simulink model "PTTransmCU"  (Simulink 7.7)
settings: Solver=ode45  StartTime=0.0  StopTime=inf  RelTol=1e-3
libraries: simulink x3, CarMaker4SL x2
(part 2 of 2)

== system PTTransmCU/CarMaker/IPG Vehicle/CarAndTrailer/Trailer/CreateBus Vhcl.Wheel.FR ==
  In1 : Inport
  Bus Creator3 : BusCreator  Inputs=14
  Demux3 : Demux  Outputs=14
  Out1 : Outport
  wires:
  Demux3/1 -> Bus Creator3/1  "Vhcl Wheel FR t x"
  Bus Creator3/1 -> Out1/1
  In1/1 -> Demux3/1
  Demux3/2 -> Bus Creator3/2  "Vhcl Wheel FR t y"
  Demux3/3 -> Bus Creator3/3  "Vhcl Wheel FR t z"
  Demux3/4 -> Bus Creator3/4  "Vhcl Wheel FR r_zxy x"
  Demux3/5 -> Bus Creator3/5  "Vhcl Wheel FR r_zxy y"
  Demux3/6 -> Bus Creator3/6  "Vhcl Wheel FR r_zxy z"
  Demux3/7 -> Bus Creator3/7  "Vhcl Wheel FR Fx"
  Demux3/8 -> Bus Creator3/8  "Vhcl Wheel FR Fy"
  Demux3/9 -> Bus Creator3/9  "Vhcl Wheel FR Fz"
  Demux3/10 -> Bus Creator3/10  "Vhcl Wheel FR vBelt"
  Demux3/11 -> Bus Creator3/11  "Vhcl Wheel FR LongSlip"
  Demux3/12 -> Bus Creator3/12  "Vhcl Wheel FR SideSlip"
  Demux3/13 -> Bus Creator3/13  "Vhcl Wheel FR Trq_T2W"
  Demux3/14 -> Bus Creator3/14  "Vhcl Wheel FR Trq_WhlBearing"

== system PTTransmCU/CarMaker/IPG Vehicle/CarAndTrailer/Trailer/CreateBus Vhcl.Wheel.RL ==
  In1 : Inport
  Bus Creator3 : BusCreator  Inputs=14
  Demux3 : Demux  Outputs=14
  Out1 : Outport
  wires:
  Demux3/1 -> Bus Creator3/1  "Vhcl Wheel RL t x"
  Bus Creator3/1 -> Out1/1
  In1/1 -> Demux3/1
  Demux3/2 -> Bus Creator3/2  "Vhcl Wheel RL t y"
  Demux3/3 -> Bus Creator3/3  "Vhcl Wheel RL t z"
  Demux3/4 -> Bus Creator3/4  "Vhcl Wheel RL r_zxy x"
  Demux3/5 -> Bus Creator3/5  "Vhcl Wheel RL r_zxy y"
  Demux3/6 -> Bus Creator3/6  "Vhcl Wheel RL r_zxy z"
  Demux3/7 -> Bus Creator3/7  "Vhcl Wheel RL Fx"
  Demux3/8 -> Bus Creator3/8  "Vhcl Wheel RL Fy"
  Demux3/9 -> Bus Creator3/9  "Vhcl Wheel RL Fz"
  Demux3/10 -> Bus Creator3/10  "Vhcl Wheel RL vBelt"
  Demux3/11 -> Bus Creator3/11  "Vhcl Wheel RL LongSlip"
  Demux3/12 -> Bus Creator3/12  "Vhcl Wheel RL SideSlip"
  Demux3/13 -> Bus Creator3/13  "Vhcl Wheel RL Trq_T2W"
  Demux3/14 -> Bus Creator3/14  "Vhcl Wheel RL Trq_WhlBearing"

== system PTTransmCU/CarMaker/IPG Vehicle/CarAndTrailer/Trailer/CreateBus Vhcl.Wheel.RR ==
  In1 : Inport
  Bus Creator3 : BusCreator  Inputs=14
  Demux3 : Demux  Outputs=14
  Out1 : Outport
  wires:
  Demux3/1 -> Bus Creator3/1  "Vhcl Wheel RR t x"
  Bus Creator3/1 -> Out1/1
  In1/1 -> Demux3/1
  Demux3/2 -> Bus Creator3/2  "Vhcl Wheel RR t y"
  Demux3/3 -> Bus Creator3/3  "Vhcl Wheel RR t z"
  Demux3/4 -> Bus Creator3/4  "Vhcl Wheel RR r_zxy x"
  Demux3/5 -> Bus Creator3/5  "Vhcl Wheel RR r_zxy y"
  Demux3/6 -> Bus Creator3/6  "Vhcl Wheel RR r_zxy z"
  Demux3/7 -> Bus Creator3/7  "Vhcl Wheel RR Fx"
  Demux3/8 -> Bus Creator3/8  "Vhcl Wheel RR Fy"
  Demux3/9 -> Bus Creator3/9  "Vhcl Wheel RR Fz"
  Demux3/10 -> Bus Creator3/10  "Vhcl Wheel RR vBelt"
  Demux3/11 -> Bus Creator3/11  "Vhcl Wheel RR LongSlip"
  Demux3/12 -> Bus Creator3/12  "Vhcl Wheel RR SideSlip"
  Demux3/13 -> Bus Creator3/13  "Vhcl Wheel RR Trq_T2W"
  Demux3/14 -> Bus Creator3/14  "Vhcl Wheel RR Trq_WhlBearing"

== system PTTransmCU/CarMaker/IPG Vehicle/PowerTrain/TCU Example/CreateBus TCU ClutchOut ==
  In : Inport
  BusCreator : BusCreator  Inputs=1
  Demux : Demux  Outputs=1
  Out : Outport
  wires:
  In/1 -> Demux/1
  BusCreator/1 -> Out/1
  Demux/1 -> BusCreator/1  "TCU ClutchOut Pos"

== system PTTransmCU/CarMaker/IPG Vehicle/PowerTrain/TCU Example/CreateBus TCU GearBoxM_Out0 ==
  In : Inport
  BusCreator : BusCreator
  Demux : Demux
  Out : Outport
  wires:
  In/1 -> Demux/1
  BusCreator/1 -> Out/1
  Demux/1 -> BusCreator/1  "TCU GearBoxM_Out0 GearNoTrg"
  Demux/2 -> BusCreator/2  "TCU GearBoxM_Out0 set_ParkBrake"
  Demux/3 -> BusCreator/3  "TCU GearBoxM_Out0 Trq_in_off"
  Demux/4 -> BusCreator/4  "TCU GearBoxM_Out0 Clutch Pos"

== system PTTransmCU/CarMaker/IPG Vehicle/PowerTrain/TCU Example/CreateBus TCU GearBoxM_Out1 ==
  In : Inport
  BusCreator : BusCreator
  Demux : Demux
  Out : Outport
  wires:
  In/1 -> Demux/1
  BusCreator/1 -> Out/1
  Demux/1 -> BusCreator/1  "TCU GearBoxM_Out1 GearNoTrg"
  Demux/2 -> BusCreator/2  "TCU GearBoxM_Out1 set_ParkBrake"
  Demux/3 -> BusCreator/3  "TCU GearBoxM_Out1 Trq_in_off"
  Demux/4 -> BusCreator/4  "TCU GearBoxM_Out1 Clutch Pos"

== system PTTransmCU/CarMaker/IPG Vehicle/PowerTrain/TCU Example/CreateBus TCU GearBoxM_Out2 ==
  In : Inport
  BusCreator : BusCreator
  Demux : Demux
  Out : Outport
  wires:
  In/1 -> Demux/1
  BusCreator/1 -> Out/1
  Demux/1 -> BusCreator/1  "TCU GearBoxM_Out2 GearNoTrg"
  Demux/2 -> BusCreator/2  "TCU GearBoxM_Out2 set_ParkBrake"
  Demux/3 -> BusCreator/3  "TCU GearBoxM_Out2 Trq_in_off"
  Demux/4 -> BusCreator/4  "TCU GearBoxM_Out2 Clutch Pos"

== system PTTransmCU/CarMaker/IPG Vehicle/PowerTrain/TCU Example/CreateBus TCU GearBoxM_Out3 ==
  In : Inport
  BusCreator : BusCreator
  Demux : Demux
  Out : Outport
  wires:
  In/1 -> Demux/1
  BusCreator/1 -> Out/1
  Demux/1 -> BusCreator/1  "TCU GearBoxM_Out3 GearNoTrg"
  Demux/2 -> BusCreator/2  "TCU GearBoxM_Out3 set_ParkBrake"
  Demux/3 -> BusCreator/3  "TCU GearBoxM_Out3 Trq_in_off"
  Demux/4 -> BusCreator/4  "TCU GearBoxM_Out3 Clutch Pos"

== system PTTransmCU/CarMaker/IPG Vehicle/PowerTrain/TCU Example/CreateBus TCU GearBoxOut ==
  In : Inport
  BusCreator : BusCreator
  Demux : Demux
  Out : Outport
  wires:
  In/1 -> Demux/1
  BusCreator/1 -> Out/1
  Demux/1 -> BusCreator/1  "TCU GearBoxOut GearNoTrg"
  Demux/2 -> BusCreator/2  "TCU GearBoxOut set_ParkBrake"
  Demux/3 -> BusCreator/3  "TCU GearBoxOut Trq_in_off"
  Demux/4 -> BusCreator/4  "TCU GearBoxOut Clutch Pos"

== system PTTransmCU/CarMaker/IPG Vehicle/PowerTrain/TCU Example/CreateBus TCU Status ==
  In : Inport
  BusCreator : BusCreator  Inputs=1
  Demux : Demux  Outputs=1
  Out : Outport
  wires:
  In/1 -> Demux/1
  BusCreator/1 -> Out/1
  Demux/1 -> BusCreator/1  "TCU_Out Status"

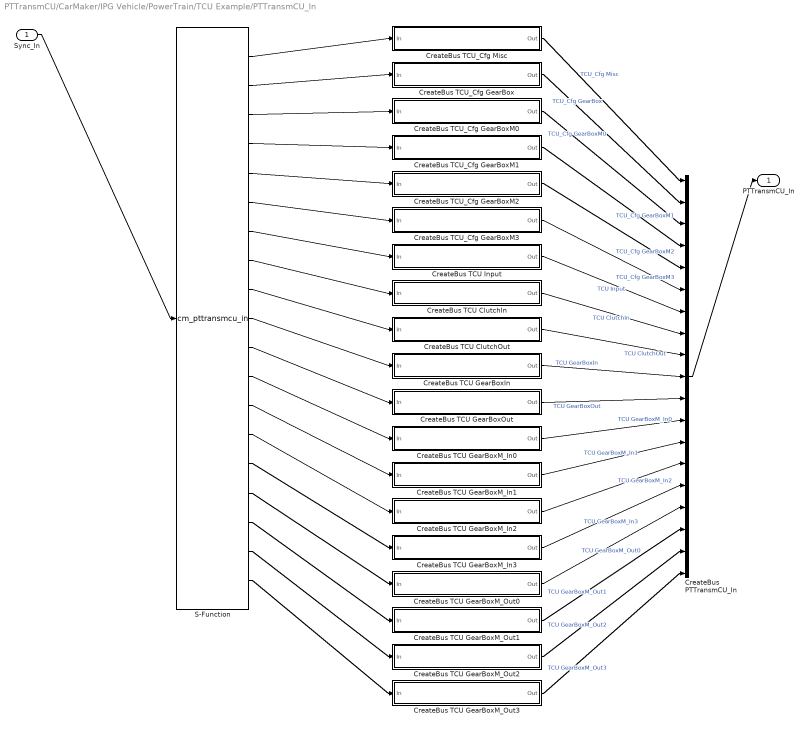
== system PTTransmCU/CarMaker/IPG Vehicle/PowerTrain/TCU Example/PTTransmCU_In ==
  Sync_In : Inport
  CreateBus PTTransmCU_In : BusCreator  Inputs=19
  CreateBus TCU ClutchIn : Subsystem
  CreateBus TCU ClutchOut : Subsystem
  CreateBus TCU GearBoxIn : Subsystem
  CreateBus TCU GearBoxM_In0 : Subsystem
  CreateBus TCU GearBoxM_In1 : Subsystem
  CreateBus TCU GearBoxM_In2 : Subsystem
  CreateBus TCU GearBoxM_In3 : Subsystem
  CreateBus TCU GearBoxM_Out0 : Subsystem
  CreateBus TCU GearBoxM_Out1 : Subsystem
  CreateBus TCU GearBoxM_Out2 : Subsystem
  CreateBus TCU GearBoxM_Out3 : Subsystem
  CreateBus TCU GearBoxOut : Subsystem
  CreateBus TCU Input : Subsystem
  CreateBus TCU_Cfg GearBox : Subsystem
  CreateBus TCU_Cfg GearBoxM0 : Subsystem
  CreateBus TCU_Cfg GearBoxM1 : Subsystem
  CreateBus TCU_Cfg GearBoxM2 : Subsystem
  CreateBus TCU_Cfg GearBoxM3 : Subsystem
  CreateBus TCU_Cfg Misc : Subsystem
  S-Function : S-Function  FunctionName=cm_pttransmcu_in  EnableBusSupport=off
  PTTransmCU_In : Outport
  wires:
  Sync_In/1 -> S-Function/1
  CreateBus PTTransmCU_In/1 -> PTTransmCU_In/1
  S-Function/1 -> CreateBus TCU_Cfg Misc/1(In)
  CreateBus TCU_Cfg Misc/1(Out) -> CreateBus PTTransmCU_In/1  "TCU_Cfg Misc"
  S-Function/2 -> CreateBus TCU_Cfg GearBox/1(In)
  CreateBus TCU_Cfg GearBox/1(Out) -> CreateBus PTTransmCU_In/2  "TCU_Cfg GearBox"
  S-Function/3 -> CreateBus TCU_Cfg GearBoxM0/1(In)
  CreateBus TCU_Cfg GearBoxM0/1(Out) -> CreateBus PTTransmCU_In/3  "TCU_Cfg GearBoxM0"
  S-Function/4 -> CreateBus TCU_Cfg GearBoxM1/1(In)
  CreateBus TCU_Cfg GearBoxM1/1(Out) -> CreateBus PTTransmCU_In/4  "TCU_Cfg GearBoxM1"
  S-Function/5 -> CreateBus TCU_Cfg GearBoxM2/1(In)
  CreateBus TCU_Cfg GearBoxM2/1(Out) -> CreateBus PTTransmCU_In/5  "TCU_Cfg GearBoxM2"
  S-Function/6 -> CreateBus TCU_Cfg GearBoxM3/1(In)
  CreateBus TCU_Cfg GearBoxM3/1(Out) -> CreateBus PTTransmCU_In/6  "TCU_Cfg GearBoxM3"
  S-Function/7 -> CreateBus TCU Input/1(In)
  CreateBus TCU Input/1(Out) -> CreateBus PTTransmCU_In/7  "TCU Input"
  S-Function/8 -> CreateBus TCU ClutchIn/1(In)
  CreateBus TCU ClutchIn/1(Out) -> CreateBus PTTransmCU_In/8  "TCU ClutchIn"
  S-Function/9 -> CreateBus TCU ClutchOut/1(In)
  CreateBus TCU ClutchOut/1(Out) -> CreateBus PTTransmCU_In/9  "TCU ClutchOut"
  S-Function/10 -> CreateBus TCU GearBoxIn/1(In)
  CreateBus TCU GearBoxIn/1(Out) -> CreateBus PTTransmCU_In/10  "TCU GearBoxIn"
  S-Function/11 -> CreateBus TCU GearBoxOut/1(In)
  CreateBus TCU GearBoxOut/1(Out) -> CreateBus PTTransmCU_In/11  "TCU GearBoxOut"
  S-Function/12 -> CreateBus TCU GearBoxM_In0/1(In)
  CreateBus TCU GearBoxM_In0/1(Out) -> CreateBus PTTransmCU_In/12  "TCU GearBoxM_In0"
  S-Function/13 -> CreateBus TCU GearBoxM_In1/1(In)
  CreateBus TCU GearBoxM_In1/1(Out) -> CreateBus PTTransmCU_In/13  "TCU GearBoxM_In1"
  S-Function/14 -> CreateBus TCU GearBoxM_In2/1(In)
  CreateBus TCU GearBoxM_In2/1(Out) -> CreateBus PTTransmCU_In/14  "TCU GearBoxM_In2"
  S-Function/15 -> CreateBus TCU GearBoxM_In3/1(In)
  CreateBus TCU GearBoxM_In3/1(Out) -> CreateBus PTTransmCU_In/15  "TCU GearBoxM_In3"
  S-Function/16 -> CreateBus TCU GearBoxM_Out0/1(In)
  CreateBus TCU GearBoxM_Out0/1(Out) -> CreateBus PTTransmCU_In/16  "TCU GearBoxM_Out0"
  S-Function/17 -> CreateBus TCU GearBoxM_Out1/1(In)
  CreateBus TCU GearBoxM_Out1/1(Out) -> CreateBus PTTransmCU_In/17  "TCU GearBoxM_Out1"
  S-Function/18 -> CreateBus TCU GearBoxM_Out2/1(In)
  CreateBus TCU GearBoxM_Out2/1(Out) -> CreateBus PTTransmCU_In/18  "TCU GearBoxM_Out2"
  S-Function/19 -> CreateBus TCU GearBoxM_Out3/1(In)
  CreateBus TCU GearBoxM_Out3/1(Out) -> CreateBus PTTransmCU_In/19  "TCU GearBoxM_Out3"

== system PTTransmCU/CarMaker/IPG Vehicle/PowerTrain/TCU Example/PTTransmCU_Out ==
  TCU Status : Inport
  TCU ClutchOut : Inport  Port=2
  TCU GearBoxOut : Inport  Port=3
  TCU GearBoxM_Out0 : Inport  Port=4
  TCU GearBoxM_Out1 : Inport  Port=5
  TCU GearBoxM_Out2 : Inport  Port=6
  TCU GearBoxM_Out3 : Inport  Port=7
  S-Function : S-Function  FunctionName=cm_pttransmcu_out  EnableBusSupport=off
  wires:
  TCU Status/1 -> S-Function/1
  TCU ClutchOut/1 -> S-Function/2
  TCU GearBoxOut/1 -> S-Function/3
  TCU GearBoxM_Out0/1 -> S-Function/4
  TCU GearBoxM_Out1/1 -> S-Function/5
  TCU GearBoxM_Out2/1 -> S-Function/6
  TCU GearBoxM_Out3/1 -> S-Function/7

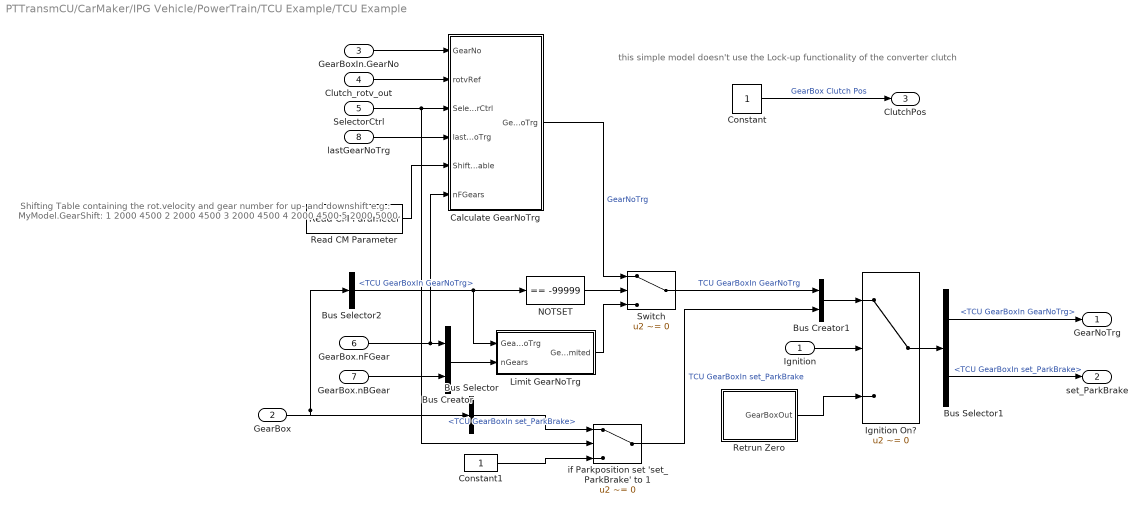
== system PTTransmCU/CarMaker/IPG Vehicle/PowerTrain/TCU Example/TCU Example ==
  note: this simple model doesn't use the
      | Lock-up functionality of the converter clutch
  note: Shifting Table containing the rot.velocity
      | and gear number for up- and downshift
      | e.g.:
      | MyModel.GearShift:
      |     1    2000    4500
      |     2    2000    4500
      |     3    2000    4500
      |     4    2000    4500
      |     5    2000    5000
  Ignition : Inport
  GearBox : Inport  Port=2
  GearBoxIn.GearNo : Inport  Port=3
  Clutch_rotv_out : Inport  Port=4
  SelectorCtrl : Inport  Port=5
  GearBox.nFGear : Inport  Port=6
  GearBox.nBGear : Inport  Port=7
  lastGearNoTrg : Inport  Port=8
  Bus Creator : BusCreator  Inputs=2
  Bus Creator1 : BusCreator  Inputs=2
  Bus Selector : BusSelector  OutputSignals=TCU GearBoxIn set_ParkBrake
  Bus Selector1 : BusSelector  OutputSignals=TCU GearBoxIn GearNoTrg,TCU GearBoxIn set_ParkBrake
  Bus Selector2 : BusSelector  OutputSignals=TCU GearBoxIn GearNoTrg
  Calculate GearNoTrg : Subsystem  TreatAsAtomicUnit=on
  Constant : Constant
  Constant1 : Constant
  Ignition On? : Switch  Criteria=u2 ~= 0
  Limit GearNoTrg : Subsystem
  NOTSET : simulink/Logic and Bit Operations/Compare To Constant  SystemSampleTime=-1  relop===  const=-99999  LogicOutDataTypeMode=uint8
  Read CM Parameter : CarMaker4SL/Read CM Parameter  xfile=Vehicle  xkey=MyModel.GearShift  xnout=80  xdefaults=0  xmuxed=on
  Retrun Zero : Subsystem  TreatAsAtomicUnit=on
  Switch : Switch  Criteria=u2 ~= 0
  if Parkposition set 'set_ParkBrake' to 1 : Switch  Criteria=u2 ~= 0
  GearNoTrg : Outport
  set_ParkBrake : Outport  Port=2
  ClutchPos : Outport  Port=3
  wires:
  GearBox/1 -> Bus Selector2/1, Bus Selector/1
  GearBox.nFGear/1 -> Bus Creator/1, Calculate GearNoTrg/6(nFGears)
  GearBoxIn.GearNo/1 -> Calculate GearNoTrg/1(GearNo)
  Constant/1 -> ClutchPos/1  "GearBox Clutch Pos"
  NOTSET/1 -> Switch/2
  Bus Selector2/1 -> Limit GearNoTrg/1(GearNoTrg), NOTSET/1  "<TCU GearBoxIn GearNoTrg>"
  Bus Creator/1 -> Limit GearNoTrg/2(nGears)
  Ignition/1 -> Ignition On?/2
  Clutch_rotv_out/1 -> Calculate GearNoTrg/2(rotvRef)
  SelectorCtrl/1 -> Calculate GearNoTrg/3(SelectorCtrl), if Parkposition set 'set_ParkBrake' to 1/2
  Read CM Parameter/1 -> Calculate GearNoTrg/5(ShiftingTable)
  Bus Creator1/1 -> Ignition On?/1
  Switch/1 -> Bus Creator1/1  "TCU GearBoxIn GearNoTrg"
  Calculate GearNoTrg/1(GearNoTrg) -> Switch/1  "GearNoTrg"
  Limit GearNoTrg/1(GearNoTrg_limited) -> Switch/3
  lastGearNoTrg/1 -> Calculate GearNoTrg/4(lastGearNoTrg)
  GearBox.nBGear/1 -> Bus Creator/2
  Bus Selector1/1 -> GearNoTrg/1  "<TCU GearBoxIn GearNoTrg>"
  Bus Selector1/2 -> set_ParkBrake/1  "<TCU GearBoxIn set_ParkBrake>"
  Retrun Zero/1(GearBoxOut) -> Ignition On?/3
  Ignition On?/1 -> Bus Selector1/1
  if Parkposition set 'set_ParkBrake' to 1/1 -> Bus Creator1/2  "TCU GearBoxIn set_ParkBrake"
  Bus Selector/1 -> if Parkposition set 'set_ParkBrake' to 1/1  "<TCU GearBoxIn set_ParkBrake>"
  Constant1/1 -> if Parkposition set 'set_ParkBrake' to 1/3

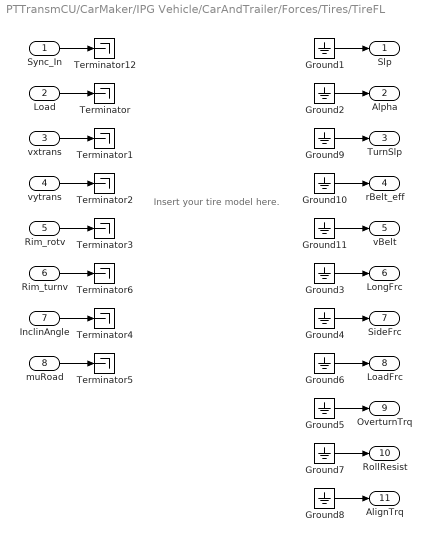
== system PTTransmCU/CarMaker/IPG Vehicle/CarAndTrailer/Forces/Tires/TireFL ==
  note: Insert your tire model here.
  Sync_In : Inport
  Load : Inport  Port=2
  vxtrans : Inport  Port=3
  vytrans : Inport  Port=4
  Rim_rotv : Inport  Port=5
  Rim_turnv : Inport  Port=6
  InclinAngle : Inport  Port=7
  muRoad : Inport  Port=8
  Ground{1..11} (11 alike) : Ground
  Terminator{,1..6,12} (8 alike) : Terminator
  Slp : Outport
  Alpha : Outport  Port=2
  TurnSlp : Outport  Port=3
  rBelt_eff : Outport  Port=4
  vBelt : Outport  Port=5
  LongFrc : Outport  Port=6
  SideFrc : Outport  Port=7
  LoadFrc : Outport  Port=8
  OverturnTrq : Outport  Port=9
  RollResist : Outport  Port=10
  AlignTrq : Outport  Port=11
  wires:
  Ground11/1 -> vBelt/1
  Ground10/1 -> rBelt_eff/1
  Ground9/1 -> TurnSlp/1
  Rim_turnv/1 -> Terminator6/1
  Sync_In/1 -> Terminator12/1
  Ground2/1 -> Alpha/1
  Ground3/1 -> LongFrc/1
  Ground4/1 -> SideFrc/1
  Ground5/1 -> OverturnTrq/1
  vxtrans/1 -> Terminator1/1
  vytrans/1 -> Terminator2/1
  Rim_rotv/1 -> Terminator3/1
  InclinAngle/1 -> Terminator4/1
  muRoad/1 -> Terminator5/1
  Load/1 -> Terminator/1
  Ground1/1 -> Slp/1
  Ground6/1 -> LoadFrc/1
  Ground7/1 -> RollResist/1
  Ground8/1 -> AlignTrq/1

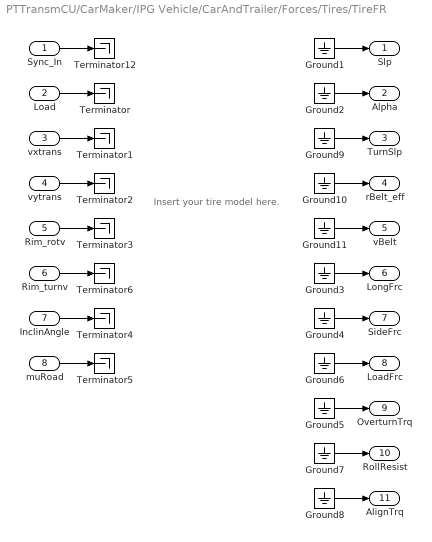
== system PTTransmCU/CarMaker/IPG Vehicle/CarAndTrailer/Forces/Tires/TireFR ==
  note: Insert your tire model here.
  Sync_In : Inport
  Load : Inport  Port=2
  vxtrans : Inport  Port=3
  vytrans : Inport  Port=4
  Rim_rotv : Inport  Port=5
  Rim_turnv : Inport  Port=6
  InclinAngle : Inport  Port=7
  muRoad : Inport  Port=8
  Ground{1..11} (11 alike) : Ground
  Terminator{,1..6,12} (8 alike) : Terminator
  Slp : Outport
  Alpha : Outport  Port=2
  TurnSlp : Outport  Port=3
  rBelt_eff : Outport  Port=4
  vBelt : Outport  Port=5
  LongFrc : Outport  Port=6
  SideFrc : Outport  Port=7
  LoadFrc : Outport  Port=8
  OverturnTrq : Outport  Port=9
  RollResist : Outport  Port=10
  AlignTrq : Outport  Port=11
  wires:
  Ground11/1 -> vBelt/1
  Ground10/1 -> rBelt_eff/1
  Ground9/1 -> TurnSlp/1
  Rim_turnv/1 -> Terminator6/1
  Sync_In/1 -> Terminator12/1
  Ground2/1 -> Alpha/1
  Ground3/1 -> LongFrc/1
  Ground4/1 -> SideFrc/1
  Ground5/1 -> OverturnTrq/1
  vxtrans/1 -> Terminator1/1
  vytrans/1 -> Terminator2/1
  Rim_rotv/1 -> Terminator3/1
  InclinAngle/1 -> Terminator4/1
  muRoad/1 -> Terminator5/1
  Load/1 -> Terminator/1
  Ground1/1 -> Slp/1
  Ground6/1 -> LoadFrc/1
  Ground7/1 -> RollResist/1
  Ground8/1 -> AlignTrq/1

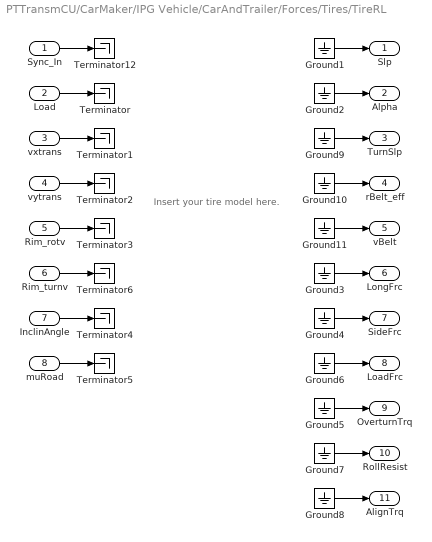
== system PTTransmCU/CarMaker/IPG Vehicle/CarAndTrailer/Forces/Tires/TireRL ==
  note: Insert your tire model here.
  Sync_In : Inport
  Load : Inport  Port=2
  vxtrans : Inport  Port=3
  vytrans : Inport  Port=4
  Rim_rotv : Inport  Port=5
  Rim_turnv : Inport  Port=6
  InclinAngle : Inport  Port=7
  muRoad : Inport  Port=8
  Ground{1..11} (11 alike) : Ground
  Terminator{,1..6,12} (8 alike) : Terminator
  Slp : Outport
  Alpha : Outport  Port=2
  TurnSlp : Outport  Port=3
  rBelt_eff : Outport  Port=4
  vBelt : Outport  Port=5
  LongFrc : Outport  Port=6
  SideFrc : Outport  Port=7
  LoadFrc : Outport  Port=8
  OverturnTrq : Outport  Port=9
  RollResist : Outport  Port=10
  AlignTrq : Outport  Port=11
  wires:
  Ground11/1 -> vBelt/1
  Ground10/1 -> rBelt_eff/1
  Ground9/1 -> TurnSlp/1
  Rim_turnv/1 -> Terminator6/1
  Sync_In/1 -> Terminator12/1
  Ground2/1 -> Alpha/1
  Ground3/1 -> LongFrc/1
  Ground4/1 -> SideFrc/1
  Ground5/1 -> OverturnTrq/1
  vxtrans/1 -> Terminator1/1
  vytrans/1 -> Terminator2/1
  Rim_rotv/1 -> Terminator3/1
  InclinAngle/1 -> Terminator4/1
  muRoad/1 -> Terminator5/1
  Load/1 -> Terminator/1
  Ground1/1 -> Slp/1
  Ground6/1 -> LoadFrc/1
  Ground7/1 -> RollResist/1
  Ground8/1 -> AlignTrq/1

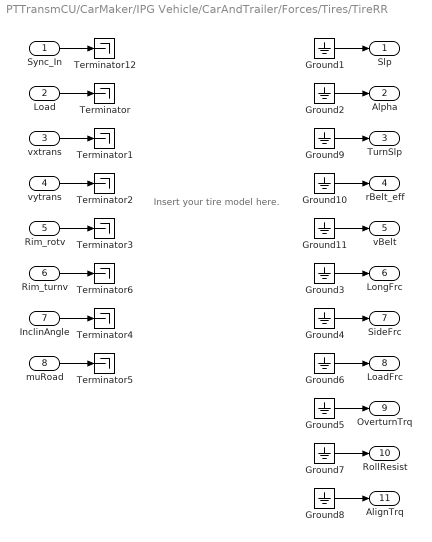
== system PTTransmCU/CarMaker/IPG Vehicle/CarAndTrailer/Forces/Tires/TireRR ==
  note: Insert your tire model here.
  Sync_In : Inport
  Load : Inport  Port=2
  vxtrans : Inport  Port=3
  vytrans : Inport  Port=4
  Rim_rotv : Inport  Port=5
  Rim_turnv : Inport  Port=6
  InclinAngle : Inport  Port=7
  muRoad : Inport  Port=8
  Ground{1..11} (11 alike) : Ground
  Terminator{,1..6,12} (8 alike) : Terminator
  Slp : Outport
  Alpha : Outport  Port=2
  TurnSlp : Outport  Port=3
  rBelt_eff : Outport  Port=4
  vBelt : Outport  Port=5
  LongFrc : Outport  Port=6
  SideFrc : Outport  Port=7
  LoadFrc : Outport  Port=8
  OverturnTrq : Outport  Port=9
  RollResist : Outport  Port=10
  AlignTrq : Outport  Port=11
  wires:
  Ground11/1 -> vBelt/1
  Ground10/1 -> rBelt_eff/1
  Ground9/1 -> TurnSlp/1
  Rim_turnv/1 -> Terminator6/1
  Sync_In/1 -> Terminator12/1
  Ground2/1 -> Alpha/1
  Ground3/1 -> LongFrc/1
  Ground4/1 -> SideFrc/1
  Ground5/1 -> OverturnTrq/1
  vxtrans/1 -> Terminator1/1
  vytrans/1 -> Terminator2/1
  Rim_rotv/1 -> Terminator3/1
  InclinAngle/1 -> Terminator4/1
  muRoad/1 -> Terminator5/1
  Load/1 -> Terminator/1
  Ground1/1 -> Slp/1
  Ground6/1 -> LoadFrc/1
  Ground7/1 -> RollResist/1
  Ground8/1 -> AlignTrq/1

== system PTTransmCU/CarMaker/IPG Vehicle/PowerTrain/TCU Example/PTTransmCU_In/CreateBus TCU ClutchIn ==
  In : Inport
  BusCreator : BusCreator  Inputs=7
  Demux : Demux  Outputs=7
  Out : Outport
  wires:
  In/1 -> Demux/1
  BusCreator/1 -> Out/1
  Demux/1 -> BusCreator/1  "TCU ClutchIn rotv_in"
  Demux/2 -> BusCreator/2  "TCU ClutchIn rotv_out"
  Demux/3 -> BusCreator/3  "TCU ClutchIn rotv_out_trg"
  Demux/4 -> BusCreator/4  "TCU ClutchIn Trq_in"
  Demux/5 -> BusCreator/5  "TCU ClutchIn Trq_out"
  Demux/6 -> BusCreator/6  "TCU ClutchIn Trq_out_trg"
  Demux/7 -> BusCreator/7  "TCU ClutchIn i_TrqIn2Out"

== system PTTransmCU/CarMaker/IPG Vehicle/PowerTrain/TCU Example/PTTransmCU_In/CreateBus TCU ClutchOut ==
  In : Inport
  BusCreator : BusCreator  Inputs=1
  Demux : Demux  Outputs=1
  Out : Outport
  wires:
  In/1 -> Demux/1
  BusCreator/1 -> Out/1
  Demux/1 -> BusCreator/1  "TCU ClutchOut Pos"

== system PTTransmCU/CarMaker/IPG Vehicle/PowerTrain/TCU Example/PTTransmCU_In/CreateBus TCU GearBoxIn ==
  In : Inport
  BusCreator : BusCreator  Inputs=15
  Demux : Demux  Outputs=15
  Out : Outport
  wires:
  In/1 -> Demux/1
  BusCreator/1 -> Out/1
  Demux/1 -> BusCreator/1  "TCU GearBoxIn GearNo"
  Demux/2 -> BusCreator/2  "TCU GearBoxIn i"
  Demux/3 -> BusCreator/3  "TCU GearBoxIn rotv_in"
  Demux/4 -> BusCreator/4  "TCU GearBoxIn rotv_in_trg"
  Demux/5 -> BusCreator/5  "TCU GearBoxIn rotv_out"
  Demux/6 -> BusCreator/6  "TCU GearBoxIn Trq_in"
  Demux/7 -> BusCreator/7  "TCU GearBoxIn Trq_out"
  Demux/8 -> BusCreator/8  "TCU GearBoxIn Trq_out_trg"
  Demux/9 -> BusCreator/9  "TCU GearBoxIn Clutch rotv_in"
  Demux/10 -> BusCreator/10  "TCU GearBoxIn Clutch rotv_out"
  Demux/11 -> BusCreator/11  "TCU GearBoxIn Clutch rotv_out_trg"
  Demux/12 -> BusCreator/12  "TCU GearBoxIn Clutch Trq_in"
  Demux/13 -> BusCreator/13  "TCU GearBoxIn Clutch Trq_out"
  Demux/14 -> BusCreator/14  "TCU GearBoxIn Clutch Trq_out_trg"
  Demux/15 -> BusCreator/15  "TCU GearBoxIn Clutch i_TrqIn2Out"

== system PTTransmCU/CarMaker/IPG Vehicle/PowerTrain/TCU Example/PTTransmCU_In/CreateBus TCU GearBoxM_In0 ==
  In : Inport
  BusCreator : BusCreator  Inputs=15
  Demux : Demux  Outputs=15
  Out : Outport
  wires:
  In/1 -> Demux/1
  BusCreator/1 -> Out/1
  Demux/1 -> BusCreator/1  "TCU GearBoxM_In0 GearNo"
  Demux/2 -> BusCreator/2  "TCU GearBoxM_In0 i"
  Demux/3 -> BusCreator/3  "TCU GearBoxM_In0 rotv_in"
  Demux/4 -> BusCreator/4  "TCU GearBoxM_In0 rotv_in_trg"
  Demux/5 -> BusCreator/5  "TCU GearBoxM_In0 rotv_out"
  Demux/6 -> BusCreator/6  "TCU GearBoxM_In0 Trq_in"
  Demux/7 -> BusCreator/7  "TCU GearBoxM_In0 Trq_out"
  Demux/8 -> BusCreator/8  "TCU GearBoxM_In0 Trq_out_trg"
  Demux/9 -> BusCreator/9  "TCU GearBoxM_In0 Clutch rotv_in"
  Demux/10 -> BusCreator/10  "TCU GearBoxM_In0 Clutch rotv_out"
  Demux/11 -> BusCreator/11  "TCU GearBoxM_In0 Clutch rotv_out_trg"
  Demux/12 -> BusCreator/12  "TCU GearBoxM_In0 Clutch Trq_in"
  Demux/13 -> BusCreator/13  "TCU GearBoxM_In0 Clutch Trq_out"
  Demux/14 -> BusCreator/14  "TCU GearBoxM_In0 Clutch Trq_out_trg"
  Demux/15 -> BusCreator/15  "TCU GearBoxM_In0 Clutch i_TrqIn2Out"

== system PTTransmCU/CarMaker/IPG Vehicle/PowerTrain/TCU Example/PTTransmCU_In/CreateBus TCU GearBoxM_In1 ==
  In : Inport
  BusCreator : BusCreator  Inputs=15
  Demux : Demux  Outputs=15
  Out : Outport
  wires:
  In/1 -> Demux/1
  BusCreator/1 -> Out/1
  Demux/1 -> BusCreator/1  "TCU GearBoxM_In1 GearNo"
  Demux/2 -> BusCreator/2  "TCU GearBoxM_In1 i"
  Demux/3 -> BusCreator/3  "TCU GearBoxM_In1 rotv_in"
  Demux/4 -> BusCreator/4  "TCU GearBoxM_In1 rotv_in_trg"
  Demux/5 -> BusCreator/5  "TCU GearBoxM_In1 rotv_out"
  Demux/6 -> BusCreator/6  "TCU GearBoxM_In1 Trq_in"
  Demux/7 -> BusCreator/7  "TCU GearBoxM_In1 Trq_out"
  Demux/8 -> BusCreator/8  "TCU GearBoxM_In1 Trq_out_trg"
  Demux/9 -> BusCreator/9  "TCU GearBoxM_In1 Clutch rotv_in"
  Demux/10 -> BusCreator/10  "TCU GearBoxM_In1 Clutch rotv_out"
  Demux/11 -> BusCreator/11  "TCU GearBoxM_In1 Clutch rotv_out_trg"
  Demux/12 -> BusCreator/12  "TCU GearBoxM_In1 Clutch Trq_in"
  Demux/13 -> BusCreator/13  "TCU GearBoxM_In1 Clutch Trq_out"
  Demux/14 -> BusCreator/14  "TCU GearBoxM_In1 Clutch Trq_out_trg"
  Demux/15 -> BusCreator/15  "TCU GearBoxM_In1 Clutch i_TrqIn2Out"

== system PTTransmCU/CarMaker/IPG Vehicle/PowerTrain/TCU Example/PTTransmCU_In/CreateBus TCU GearBoxM_In2 ==
  In : Inport
  BusCreator : BusCreator  Inputs=15
  Demux : Demux  Outputs=15
  Out : Outport
  wires:
  In/1 -> Demux/1
  BusCreator/1 -> Out/1
  Demux/1 -> BusCreator/1  "TCU GearBoxM_In2 GearNo"
  Demux/2 -> BusCreator/2  "TCU GearBoxM_In2 i"
  Demux/3 -> BusCreator/3  "TCU GearBoxM_In2 rotv_in"
  Demux/4 -> BusCreator/4  "TCU GearBoxM_In2 rotv_in_trg"
  Demux/5 -> BusCreator/5  "TCU GearBoxM_In2 rotv_out"
  Demux/6 -> BusCreator/6  "TCU GearBoxM_In2 Trq_in"
  Demux/7 -> BusCreator/7  "TCU GearBoxM_In2 Trq_out"
  Demux/8 -> BusCreator/8  "TCU GearBoxM_In2 Trq_out_trg"
  Demux/9 -> BusCreator/9  "TCU GearBoxM_In2 Clutch rotv_in"
  Demux/10 -> BusCreator/10  "TCU GearBoxM_In2 Clutch rotv_out"
  Demux/11 -> BusCreator/11  "TCU GearBoxM_In2 Clutch rotv_out_trg"
  Demux/12 -> BusCreator/12  "TCU GearBoxM_In2 Clutch Trq_in"
  Demux/13 -> BusCreator/13  "TCU GearBoxM_In2 Clutch Trq_out"
  Demux/14 -> BusCreator/14  "TCU GearBoxM_In2 Clutch Trq_out_trg"
  Demux/15 -> BusCreator/15  "TCU GearBoxM_In2 Clutch i_TrqIn2Out"

== system PTTransmCU/CarMaker/IPG Vehicle/PowerTrain/TCU Example/PTTransmCU_In/CreateBus TCU GearBoxM_In3 ==
  In : Inport
  BusCreator : BusCreator  Inputs=15
  Demux : Demux  Outputs=15
  Out : Outport
  wires:
  In/1 -> Demux/1
  BusCreator/1 -> Out/1
  Demux/1 -> BusCreator/1  "TCU GearBoxM_In3 GearNo"
  Demux/2 -> BusCreator/2  "TCU GearBoxM_In3 i"
  Demux/3 -> BusCreator/3  "TCU GearBoxM_In3 rotv_in"
  Demux/4 -> BusCreator/4  "TCU GearBoxM_In3 rotv_in_trg"
  Demux/5 -> BusCreator/5  "TCU GearBoxM_In3 rotv_out"
  Demux/6 -> BusCreator/6  "TCU GearBoxM_In3 Trq_in"
  Demux/7 -> BusCreator/7  "TCU GearBoxM_In3 Trq_out"
  Demux/8 -> BusCreator/8  "TCU GearBoxM_In3 Trq_out_trg"
  Demux/9 -> BusCreator/9  "TCU GearBoxM_In3 Clutch rotv_in"
  Demux/10 -> BusCreator/10  "TCU GearBoxM_In3 Clutch rotv_out"
  Demux/11 -> BusCreator/11  "TCU GearBoxM_In3 Clutch rotv_out_trg"
  Demux/12 -> BusCreator/12  "TCU GearBoxM_In3 Clutch Trq_in"
  Demux/13 -> BusCreator/13  "TCU GearBoxM_In3 Clutch Trq_out"
  Demux/14 -> BusCreator/14  "TCU GearBoxM_In3 Clutch Trq_out_trg"
  Demux/15 -> BusCreator/15  "TCU GearBoxM_In3 Clutch i_TrqIn2Out"

== system PTTransmCU/CarMaker/IPG Vehicle/PowerTrain/TCU Example/PTTransmCU_In/CreateBus TCU GearBoxM_Out0 ==
  In : Inport
  BusCreator : BusCreator  Inputs=3
  Demux : Demux  Outputs=3
  Out : Outport
  wires:
  In/1 -> Demux/1
  BusCreator/1 -> Out/1
  Demux/1 -> BusCreator/1  "TCU GearBoxM_Out0 GearNoTrg"
  Demux/2 -> BusCreator/2  "TCU GearBoxM_Out0 set_ParkBrake"
  Demux/3 -> BusCreator/3  "TCU GearBoxM_Out0 Clutch Pos"

== system PTTransmCU/CarMaker/IPG Vehicle/PowerTrain/TCU Example/PTTransmCU_In/CreateBus TCU GearBoxM_Out1 ==
  In : Inport
  BusCreator : BusCreator  Inputs=3
  Demux : Demux  Outputs=3
  Out : Outport
  wires:
  In/1 -> Demux/1
  BusCreator/1 -> Out/1
  Demux/1 -> BusCreator/1  "TCU GearBoxM_Out1 GearNoTrg"
  Demux/2 -> BusCreator/2  "TCU GearBoxM_Out1 set_ParkBrake"
  Demux/3 -> BusCreator/3  "TCU GearBoxM_Out1 Clutch Pos"

== system PTTransmCU/CarMaker/IPG Vehicle/PowerTrain/TCU Example/PTTransmCU_In/CreateBus TCU GearBoxM_Out2 ==
  In : Inport
  BusCreator : BusCreator  Inputs=3
  Demux : Demux  Outputs=3
  Out : Outport
  wires:
  In/1 -> Demux/1
  BusCreator/1 -> Out/1
  Demux/1 -> BusCreator/1  "TCU GearBoxM_Out2 GearNoTrg"
  Demux/2 -> BusCreator/2  "TCU GearBoxM_Out2 set_ParkBrake"
  Demux/3 -> BusCreator/3  "TCU GearBoxM_Out2 Clutch Pos"

== system PTTransmCU/CarMaker/IPG Vehicle/PowerTrain/TCU Example/PTTransmCU_In/CreateBus TCU GearBoxM_Out3 ==
  In : Inport
  BusCreator : BusCreator  Inputs=3
  Demux : Demux  Outputs=3
  Out : Outport
  wires:
  In/1 -> Demux/1
  BusCreator/1 -> Out/1
  Demux/1 -> BusCreator/1  "TCU GearBoxM_Out3 GearNoTrg"
  Demux/2 -> BusCreator/2  "TCU GearBoxM_Out3 set_ParkBrake"
  Demux/3 -> BusCreator/3  "TCU GearBoxM_Out3 Clutch Pos"

== system PTTransmCU/CarMaker/IPG Vehicle/PowerTrain/TCU Example/PTTransmCU_In/CreateBus TCU GearBoxOut ==
  In : Inport
  BusCreator : BusCreator  Inputs=3
  Demux : Demux  Outputs=3
  Out : Outport
  wires:
  In/1 -> Demux/1
  BusCreator/1 -> Out/1
  Demux/1 -> BusCreator/1  "TCU GearBoxIn GearNoTrg"
  Demux/2 -> BusCreator/2  "TCU GearBoxIn set_ParkBrake"
  Demux/3 -> BusCreator/3  "TCU GearBoxIn Clutch Pos"

== system PTTransmCU/CarMaker/IPG Vehicle/PowerTrain/TCU Example/PTTransmCU_In/CreateBus TCU Input ==
  In : Inport
  BusCreator : BusCreator  Inputs=3
  Demux : Demux  Outputs=3
  Out : Outport
  wires:
  In/1 -> Demux/1
  BusCreator/1 -> Out/1
  Demux/1 -> BusCreator/1  "TCU Ignition"
  Demux/2 -> BusCreator/2  "TCU Load"
  Demux/3 -> BusCreator/3  "TCU SelectorCtrl"

== system PTTransmCU/CarMaker/IPG Vehicle/PowerTrain/TCU Example/PTTransmCU_In/CreateBus TCU_Cfg GearBox ==
  In : Inport
  BusCreator : BusCreator  Inputs=38
  Demux : Demux  Outputs=38
  Out : Outport
  wires:
  In/1 -> Demux/1
  BusCreator/1 -> Out/1
  Demux/1 -> BusCreator/1  "TCU_Cfg GearBox GBKind"
  Demux/2 -> BusCreator/2  "TCU_Cfg GearBox ClKind"
  Demux/3 -> BusCreator/3  "TCU_Cfg GearBox nFGears"
  Demux/4 -> BusCreator/4  "TCU_Cfg GearBox iFGear0"
  Demux/5 -> BusCreator/5  "TCU_Cfg GearBox iFGear1"
  Demux/6 -> BusCreator/6  "TCU_Cfg GearBox iFGear2"
  Demux/7 -> BusCreator/7  "TCU_Cfg GearBox iFGear3"
  Demux/8 -> BusCreator/8  "TCU_Cfg GearBox iFGear4"
  Demux/9 -> BusCreator/9  "TCU_Cfg GearBox iFGear5"
  Demux/10 -> BusCreator/10  "TCU_Cfg GearBox iFGear6"
  Demux/11 -> BusCreator/11  "TCU_Cfg GearBox iFGear7"
  Demux/12 -> BusCreator/12  "TCU_Cfg GearBox iFGear8"
  Demux/13 -> BusCreator/13  "TCU_Cfg GearBox iFGear9"
  Demux/14 -> BusCreator/14  "TCU_Cfg GearBox iFGear10"
  Demux/15 -> BusCreator/15  "TCU_Cfg GearBox iFGear11"
  Demux/16 -> BusCreator/16  "TCU_Cfg GearBox iFGear12"
  Demux/17 -> BusCreator/17  "TCU_Cfg GearBox iFGear13"
  Demux/18 -> BusCreator/18  "TCU_Cfg GearBox iFGear14"
  Demux/19 -> BusCreator/19  "TCU_Cfg GearBox iFGear15"
  Demux/20 -> BusCreator/20  "TCU_Cfg GearBox iFGear16"
  Demux/21 -> BusCreator/21  "TCU_Cfg GearBox nBGears"
  Demux/22 -> BusCreator/22  "TCU_Cfg GearBox iBGear0"
  Demux/23 -> BusCreator/23  "TCU_Cfg GearBox iBGear1"
  Demux/24 -> BusCreator/24  "TCU_Cfg GearBox iBGear2"
  Demux/25 -> BusCreator/25  "TCU_Cfg GearBox iBGear3"
  Demux/26 -> BusCreator/26  "TCU_Cfg GearBox iBGear4"
  Demux/27 -> BusCreator/27  "TCU_Cfg GearBox iBGear5"
  Demux/28 -> BusCreator/28  "TCU_Cfg GearBox iBGear6"
  Demux/29 -> BusCreator/29  "TCU_Cfg GearBox iBGear7"
  Demux/30 -> BusCreator/30  "TCU_Cfg GearBox iBGear8"
  Demux/31 -> BusCreator/31  "TCU_Cfg GearBox iBGear9"
  Demux/32 -> BusCreator/32  "TCU_Cfg GearBox iBGear10"
  Demux/33 -> BusCreator/33  "TCU_Cfg GearBox iBGear11"
  Demux/34 -> BusCreator/34  "TCU_Cfg GearBox iBGear12"
  Demux/35 -> BusCreator/35  "TCU_Cfg GearBox iBGear13"
  Demux/36 -> BusCreator/36  "TCU_Cfg GearBox iBGear14"
  Demux/37 -> BusCreator/37  "TCU_Cfg GearBox iBGear15"
  Demux/38 -> BusCreator/38  "TCU_Cfg GearBox iBGear16"

== system PTTransmCU/CarMaker/IPG Vehicle/PowerTrain/TCU Example/PTTransmCU_In/CreateBus TCU_Cfg GearBoxM0 ==
  In : Inport
  BusCreator : BusCreator  Inputs=38
  Demux : Demux  Outputs=38
  Out : Outport
  wires:
  In/1 -> Demux/1
  BusCreator/1 -> Out/1
  Demux/1 -> BusCreator/1  "TCU_Cfg GearBoxM0 GBKind"
  Demux/2 -> BusCreator/2  "TCU_Cfg GearBoxM0 ClKind"
  Demux/3 -> BusCreator/3  "TCU_Cfg GearBoxM0 nFGears"
  Demux/4 -> BusCreator/4  "TCU_Cfg GearBoxM0 iFGear0"
  Demux/5 -> BusCreator/5  "TCU_Cfg GearBoxM0 iFGear1"
  Demux/6 -> BusCreator/6  "TCU_Cfg GearBoxM0 iFGear2"
  Demux/7 -> BusCreator/7  "TCU_Cfg GearBoxM0 iFGear3"
  Demux/8 -> BusCreator/8  "TCU_Cfg GearBoxM0 iFGear4"
  Demux/9 -> BusCreator/9  "TCU_Cfg GearBoxM0 iFGear5"
  Demux/10 -> BusCreator/10  "TCU_Cfg GearBoxM0 iFGear6"
  Demux/11 -> BusCreator/11  "TCU_Cfg GearBoxM0 iFGear7"
  Demux/12 -> BusCreator/12  "TCU_Cfg GearBoxM0 iFGear8"
  Demux/13 -> BusCreator/13  "TCU_Cfg GearBoxM0 iFGear9"
  Demux/14 -> BusCreator/14  "TCU_Cfg GearBoxM0 iFGear10"
  Demux/15 -> BusCreator/15  "TCU_Cfg GearBoxM0 iFGear11"
  Demux/16 -> BusCreator/16  "TCU_Cfg GearBoxM0 iFGear12"
  Demux/17 -> BusCreator/17  "TCU_Cfg GearBoxM0 iFGear13"
  Demux/18 -> BusCreator/18  "TCU_Cfg GearBoxM0 iFGear14"
  Demux/19 -> BusCreator/19  "TCU_Cfg GearBoxM0 iFGear15"
  Demux/20 -> BusCreator/20  "TCU_Cfg GearBoxM0 iFGear16"
  Demux/21 -> BusCreator/21  "TCU_Cfg GearBoxM0 nBGears"
  Demux/22 -> BusCreator/22  "TCU_Cfg GearBoxM0 iBGear0"
  Demux/23 -> BusCreator/23  "TCU_Cfg GearBoxM0 iBGear1"
  Demux/24 -> BusCreator/24  "TCU_Cfg GearBoxM0 iBGear2"
  Demux/25 -> BusCreator/25  "TCU_Cfg GearBoxM0 iBGear3"
  Demux/26 -> BusCreator/26  "TCU_Cfg GearBoxM0 iBGear4"
  Demux/27 -> BusCreator/27  "TCU_Cfg GearBoxM0 iBGear5"
  Demux/28 -> BusCreator/28  "TCU_Cfg GearBoxM0 iBGear6"
  Demux/29 -> BusCreator/29  "TCU_Cfg GearBoxM0 iBGear7"
  Demux/30 -> BusCreator/30  "TCU_Cfg GearBoxM0 iBGear8"
  Demux/31 -> BusCreator/31  "TCU_Cfg GearBoxM0 iBGear9"
  Demux/32 -> BusCreator/32  "TCU_Cfg GearBoxM0 iBGear10"
  Demux/33 -> BusCreator/33  "TCU_Cfg GearBoxM0 iBGear11"
  Demux/34 -> BusCreator/34  "TCU_Cfg GearBoxM0 iBGear12"
  Demux/35 -> BusCreator/35  "TCU_Cfg GearBoxM0 iBGear13"
  Demux/36 -> BusCreator/36  "TCU_Cfg GearBoxM0 iBGear14"
  Demux/37 -> BusCreator/37  "TCU_Cfg GearBoxM0 iBGear15"
  Demux/38 -> BusCreator/38  "TCU_Cfg GearBoxM0 iBGear16"

== system PTTransmCU/CarMaker/IPG Vehicle/PowerTrain/TCU Example/PTTransmCU_In/CreateBus TCU_Cfg GearBoxM1 ==
  In : Inport
  BusCreator : BusCreator  Inputs=38
  Demux : Demux  Outputs=38
  Out : Outport
  wires:
  In/1 -> Demux/1
  BusCreator/1 -> Out/1
  Demux/1 -> BusCreator/1  "TCU_Cfg GearBoxM1 GBKind"
  Demux/2 -> BusCreator/2  "TCU_Cfg GearBoxM1 ClKind"
  Demux/3 -> BusCreator/3  "TCU_Cfg GearBoxM1 nFGears"
  Demux/4 -> BusCreator/4  "TCU_Cfg GearBoxM1 iFGear0"
  Demux/5 -> BusCreator/5  "TCU_Cfg GearBoxM1 iFGear1"
  Demux/6 -> BusCreator/6  "TCU_Cfg GearBoxM1 iFGear2"
  Demux/7 -> BusCreator/7  "TCU_Cfg GearBoxM1 iFGear3"
  Demux/8 -> BusCreator/8  "TCU_Cfg GearBoxM1 iFGear4"
  Demux/9 -> BusCreator/9  "TCU_Cfg GearBoxM1 iFGear5"
  Demux/10 -> BusCreator/10  "TCU_Cfg GearBoxM1 iFGear6"
  Demux/11 -> BusCreator/11  "TCU_Cfg GearBoxM1 iFGear7"
  Demux/12 -> BusCreator/12  "TCU_Cfg GearBoxM1 iFGear8"
  Demux/13 -> BusCreator/13  "TCU_Cfg GearBoxM1 iFGear9"
  Demux/14 -> BusCreator/14  "TCU_Cfg GearBoxM1 iFGear10"
  Demux/15 -> BusCreator/15  "TCU_Cfg GearBoxM1 iFGear11"
  Demux/16 -> BusCreator/16  "TCU_Cfg GearBoxM1 iFGear12"
  Demux/17 -> BusCreator/17  "TCU_Cfg GearBoxM1 iFGear13"
  Demux/18 -> BusCreator/18  "TCU_Cfg GearBoxM1 iFGear14"
  Demux/19 -> BusCreator/19  "TCU_Cfg GearBoxM1 iFGear15"
  Demux/20 -> BusCreator/20  "TCU_Cfg GearBoxM1 iFGear16"
  Demux/21 -> BusCreator/21  "TCU_Cfg GearBoxM1 nBGears"
  Demux/22 -> BusCreator/22  "TCU_Cfg GearBoxM1 iBGear0"
  Demux/23 -> BusCreator/23  "TCU_Cfg GearBoxM1 iBGear1"
  Demux/24 -> BusCreator/24  "TCU_Cfg GearBoxM1 iBGear2"
  Demux/25 -> BusCreator/25  "TCU_Cfg GearBoxM1 iBGear3"
  Demux/26 -> BusCreator/26  "TCU_Cfg GearBoxM1 iBGear4"
  Demux/27 -> BusCreator/27  "TCU_Cfg GearBoxM1 iBGear5"
  Demux/28 -> BusCreator/28  "TCU_Cfg GearBoxM1 iBGear6"
  Demux/29 -> BusCreator/29  "TCU_Cfg GearBoxM1 iBGear7"
  Demux/30 -> BusCreator/30  "TCU_Cfg GearBoxM1 iBGear8"
  Demux/31 -> BusCreator/31  "TCU_Cfg GearBoxM1 iBGear9"
  Demux/32 -> BusCreator/32  "TCU_Cfg GearBoxM1 iBGear10"
  Demux/33 -> BusCreator/33  "TCU_Cfg GearBoxM1 iBGear11"
  Demux/34 -> BusCreator/34  "TCU_Cfg GearBoxM1 iBGear12"
  Demux/35 -> BusCreator/35  "TCU_Cfg GearBoxM1 iBGear13"
  Demux/36 -> BusCreator/36  "TCU_Cfg GearBoxM1 iBGear14"
  Demux/37 -> BusCreator/37  "TCU_Cfg GearBoxM1 iBGear15"
  Demux/38 -> BusCreator/38  "TCU_Cfg GearBoxM1 iBGear16"

== system PTTransmCU/CarMaker/IPG Vehicle/PowerTrain/TCU Example/PTTransmCU_In/CreateBus TCU_Cfg GearBoxM2 ==
  In : Inport
  BusCreator : BusCreator  Inputs=38
  Demux : Demux  Outputs=38
  Out : Outport
  wires:
  In/1 -> Demux/1
  BusCreator/1 -> Out/1
  Demux/1 -> BusCreator/1  "TCU_Cfg GearBoxM2 GBKind"
  Demux/2 -> BusCreator/2  "TCU_Cfg GearBoxM2 ClKind"
  Demux/3 -> BusCreator/3  "TCU_Cfg GearBoxM2 nFGears"
  Demux/4 -> BusCreator/4  "TCU_Cfg GearBoxM2 iFGear0"
  Demux/5 -> BusCreator/5  "TCU_Cfg GearBoxM2 iFGear1"
  Demux/6 -> BusCreator/6  "TCU_Cfg GearBoxM2 iFGear2"
  Demux/7 -> BusCreator/7  "TCU_Cfg GearBoxM2 iFGear3"
  Demux/8 -> BusCreator/8  "TCU_Cfg GearBoxM2 iFGear4"
  Demux/9 -> BusCreator/9  "TCU_Cfg GearBoxM2 iFGear5"
  Demux/10 -> BusCreator/10  "TCU_Cfg GearBoxM2 iFGear6"
  Demux/11 -> BusCreator/11  "TCU_Cfg GearBoxM2 iFGear7"
  Demux/12 -> BusCreator/12  "TCU_Cfg GearBoxM2 iFGear8"
  Demux/13 -> BusCreator/13  "TCU_Cfg GearBoxM2 iFGear9"
  Demux/14 -> BusCreator/14  "TCU_Cfg GearBoxM2 iFGear10"
  Demux/15 -> BusCreator/15  "TCU_Cfg GearBoxM2 iFGear11"
  Demux/16 -> BusCreator/16  "TCU_Cfg GearBoxM2 iFGear12"
  Demux/17 -> BusCreator/17  "TCU_Cfg GearBoxM2 iFGear13"
  Demux/18 -> BusCreator/18  "TCU_Cfg GearBoxM2 iFGear14"
  Demux/19 -> BusCreator/19  "TCU_Cfg GearBoxM2 iFGear15"
  Demux/20 -> BusCreator/20  "TCU_Cfg GearBoxM2 iFGear16"
  Demux/21 -> BusCreator/21  "TCU_Cfg GearBoxM2 nBGears"
  Demux/22 -> BusCreator/22  "TCU_Cfg GearBoxM2 iBGear0"
  Demux/23 -> BusCreator/23  "TCU_Cfg GearBoxM2 iBGear1"
  Demux/24 -> BusCreator/24  "TCU_Cfg GearBoxM2 iBGear2"
  Demux/25 -> BusCreator/25  "TCU_Cfg GearBoxM2 iBGear3"
  Demux/26 -> BusCreator/26  "TCU_Cfg GearBoxM2 iBGear4"
  Demux/27 -> BusCreator/27  "TCU_Cfg GearBoxM2 iBGear5"
  Demux/28 -> BusCreator/28  "TCU_Cfg GearBoxM2 iBGear6"
  Demux/29 -> BusCreator/29  "TCU_Cfg GearBoxM2 iBGear7"
  Demux/30 -> BusCreator/30  "TCU_Cfg GearBoxM2 iBGear8"
  Demux/31 -> BusCreator/31  "TCU_Cfg GearBoxM2 iBGear9"
  Demux/32 -> BusCreator/32  "TCU_Cfg GearBoxM2 iBGear10"
  Demux/33 -> BusCreator/33  "TCU_Cfg GearBoxM2 iBGear11"
  Demux/34 -> BusCreator/34  "TCU_Cfg GearBoxM2 iBGear12"
  Demux/35 -> BusCreator/35  "TCU_Cfg GearBoxM2 iBGear13"
  Demux/36 -> BusCreator/36  "TCU_Cfg GearBoxM2 iBGear14"
  Demux/37 -> BusCreator/37  "TCU_Cfg GearBoxM2 iBGear15"
  Demux/38 -> BusCreator/38  "TCU_Cfg GearBoxM2 iBGear16"

== system PTTransmCU/CarMaker/IPG Vehicle/PowerTrain/TCU Example/PTTransmCU_In/CreateBus TCU_Cfg GearBoxM3 ==
  In : Inport
  BusCreator : BusCreator  Inputs=38
  Demux : Demux  Outputs=38
  Out : Outport
  wires:
  In/1 -> Demux/1
  BusCreator/1 -> Out/1
  Demux/1 -> BusCreator/1  "TCU_Cfg GearBoxM3 GBKind"
  Demux/2 -> BusCreator/2  "TCU_Cfg GearBoxM3 ClKind"
  Demux/3 -> BusCreator/3  "TCU_Cfg GearBoxM3 nFGears"
  Demux/4 -> BusCreator/4  "TCU_Cfg GearBoxM3 iFGear0"
  Demux/5 -> BusCreator/5  "TCU_Cfg GearBoxM3 iFGear1"
  Demux/6 -> BusCreator/6  "TCU_Cfg GearBoxM3 iFGear2"
  Demux/7 -> BusCreator/7  "TCU_Cfg GearBoxM3 iFGear3"
  Demux/8 -> BusCreator/8  "TCU_Cfg GearBoxM3 iFGear4"
  Demux/9 -> BusCreator/9  "TCU_Cfg GearBoxM3 iFGear5"
  Demux/10 -> BusCreator/10  "TCU_Cfg GearBoxM3 iFGear6"
  Demux/11 -> BusCreator/11  "TCU_Cfg GearBoxM3 iFGear7"
  Demux/12 -> BusCreator/12  "TCU_Cfg GearBoxM3 iFGear8"
  Demux/13 -> BusCreator/13  "TCU_Cfg GearBoxM3 iFGear9"
  Demux/14 -> BusCreator/14  "TCU_Cfg GearBoxM3 iFGear10"
  Demux/15 -> BusCreator/15  "TCU_Cfg GearBoxM3 iFGear11"
  Demux/16 -> BusCreator/16  "TCU_Cfg GearBoxM3 iFGear12"
  Demux/17 -> BusCreator/17  "TCU_Cfg GearBoxM3 iFGear13"
  Demux/18 -> BusCreator/18  "TCU_Cfg GearBoxM3 iFGear14"
  Demux/19 -> BusCreator/19  "TCU_Cfg GearBoxM3 iFGear15"
  Demux/20 -> BusCreator/20  "TCU_Cfg GearBoxM3 iFGear16"
  Demux/21 -> BusCreator/21  "TCU_Cfg GearBoxM3 nBGears"
  Demux/22 -> BusCreator/22  "TCU_Cfg GearBoxM3 iBGear0"
  Demux/23 -> BusCreator/23  "TCU_Cfg GearBoxM3 iBGear1"
  Demux/24 -> BusCreator/24  "TCU_Cfg GearBoxM3 iBGear2"
  Demux/25 -> BusCreator/25  "TCU_Cfg GearBoxM3 iBGear3"
  Demux/26 -> BusCreator/26  "TCU_Cfg GearBoxM3 iBGear4"
  Demux/27 -> BusCreator/27  "TCU_Cfg GearBoxM3 iBGear5"
  Demux/28 -> BusCreator/28  "TCU_Cfg GearBoxM3 iBGear6"
  Demux/29 -> BusCreator/29  "TCU_Cfg GearBoxM3 iBGear7"
  Demux/30 -> BusCreator/30  "TCU_Cfg GearBoxM3 iBGear8"
  Demux/31 -> BusCreator/31  "TCU_Cfg GearBoxM3 iBGear9"
  Demux/32 -> BusCreator/32  "TCU_Cfg GearBoxM3 iBGear10"
  Demux/33 -> BusCreator/33  "TCU_Cfg GearBoxM3 iBGear11"
  Demux/34 -> BusCreator/34  "TCU_Cfg GearBoxM3 iBGear12"
  Demux/35 -> BusCreator/35  "TCU_Cfg GearBoxM3 iBGear13"
  Demux/36 -> BusCreator/36  "TCU_Cfg GearBoxM3 iBGear14"
  Demux/37 -> BusCreator/37  "TCU_Cfg GearBoxM3 iBGear15"
  Demux/38 -> BusCreator/38  "TCU_Cfg GearBoxM3 iBGear16"

== system PTTransmCU/CarMaker/IPG Vehicle/PowerTrain/TCU Example/PTTransmCU_In/CreateBus TCU_Cfg Misc ==
  In : Inport
  BusCreator : BusCreator  Inputs=2
  Demux : Demux  Outputs=2
  Out : Outport
  wires:
  In/1 -> Demux/1
  BusCreator/1 -> Out/1
  Demux/1 -> BusCreator/1  "TCU_Cfg ClKind"
  Demux/2 -> BusCreator/2  "TCU_Cfg nGearBoxM"

== system PTTransmCU/CarMaker/IPG Vehicle/PowerTrain/TCU Example/TCU Example/Calculate GearNoTrg ==
  GearNo : Inport
  rotvRef : Inport  Port=2
  SelectorCtrl : Inport  Port=3
  lastGearNoTrg : Inport  Port=4
  ShiftingTable : Inport  Port=5
  nFGears : Inport  Port=6
  Abs : Abs
  Backwards : Subsystem  TreatAsAtomicUnit=on
  Bias : Bias  Bias=-1
  Bias1 : Bias  Bias=-2
  Constant : Constant
  Driving : Subsystem  TreatAsAtomicUnit=on
  Gain : Gain  Gain=3
  Lower Limit : MultiPortSwitch  DataPortOrder=Zero-based contiguous  Inputs=1  zeroidx=on
  Merge : Merge  Inputs=3
  Switch : Switch  Criteria=u2 ~= 0
  Switch Case : SwitchCase  CaseConditions={1,-1}
  Upper Limit : MultiPortSwitch  DataPortOrder=Zero-based contiguous  Inputs=1  zeroidx=on
  else : Subsystem  TreatAsAtomicUnit=on
  rpm2radsec : Gain  Gain=0.104719755
  rpm2radsec1 : Gain  Gain=0.104719755
  GearNoTrg : Outport
  wires:
  Upper Limit/1 -> rpm2radsec/1
  Bias/1 -> Upper Limit/1
  ShiftingTable/1 -> Upper Limit/2, Lower Limit/2
  Gain/1 -> Bias/1, Bias1/1
  Bias1/1 -> Lower Limit/1
  GearNo/1 -> Driving/1(GearNo), Switch/2, Switch/1
  Lower Limit/1 -> rpm2radsec1/1
  SelectorCtrl/1 -> Switch Case/1
  Switch Case/1 -> Driving/Action
  Driving/1(GearNoTrg) -> Merge/1
  Backwards/1(GearNoTrg) -> Merge/2
  else/1(GearNoTrg) -> Merge/3
  Merge/1 -> GearNoTrg/1
  Switch Case/2 -> Backwards/Action
  Switch Case/3 -> else/Action
  Abs/1 -> Gain/1
  rotvRef/1 -> Driving/4(rotvRef)
  rpm2radsec/1 -> Driving/2(Upper Limit)
  rpm2radsec1/1 -> Driving/3(Lower Limit)
  nFGears/1 -> Driving/5(nFGears)
  lastGearNoTrg/1 -> Driving/6(GearNoTrg_last)
  Switch/1 -> Abs/1
  Constant/1 -> Switch/3

== system PTTransmCU/CarMaker/IPG Vehicle/PowerTrain/TCU Example/TCU Example/Limit GearNoTrg ==
  GearNoTrg : Inport
  nGears : Inport  Port=2
  Bus Selector : BusSelector  OutputSignals=TCU_Cfg GearBox nFGears,TCU_Cfg GearBox nBGears
  Gain : Gain  Gain=-1
  Saturation Dynamic : simulink/Discontinuities/Saturation Dynamic  SystemSampleTime=-1  OutMin=[]  OutMax=[]  OutDataTypeStr=Inherit: Same as second input  OutDataType=sfix(16)  OutScaling=2^-10  DoSatur=off
  GearNoTrg_limited : Outport
  wires:
  GearNoTrg/1 -> Saturation Dynamic/2
  Bus Selector/1 -> Saturation Dynamic/1  "<TCU_Cfg GearBox nFGears>"
  Bus Selector/2 -> Gain/1  "<TCU_Cfg GearBox nBGears>"
  Gain/1 -> Saturation Dynamic/3
  Saturation Dynamic/1 -> GearNoTrg_limited/1
  nGears/1 -> Bus Selector/1

== system PTTransmCU/CarMaker/IPG Vehicle/PowerTrain/TCU Example/TCU Example/Retrun Zero ==
  Bus Creator : BusCreator  Inputs=2
  Constant : Constant  Value=0
  Constant1 : Constant  Value=0
  GearBoxOut : Outport
  wires:
  Constant/1 -> Bus Creator/1  "TCU GearBoxIn GearNoTrg"
  Constant1/1 -> Bus Creator/2  "TCU GearBoxIn set_ParkBrake"
  Bus Creator/1 -> GearBoxOut/1

== system PTTransmCU/CarMaker/IPG Vehicle/PowerTrain/TCU Example/TCU Example/Calculate GearNoTrg/Backwards ==
  Action Port : ActionPort  ActionType=case
  Constant : Constant  Value=-1
  GearNoTrg : Outport  InitialOutput=-1
  wires:
  Constant/1 -> GearNoTrg/1

== system PTTransmCU/CarMaker/IPG Vehicle/PowerTrain/TCU Example/TCU Example/Calculate GearNoTrg/Driving ==
  GearNo : Inport
  Upper Limit : Inport  Port=2
  Lower Limit : Inport  Port=3
  rotvRef : Inport  Port=4
  nFGears : Inport  Port=5
  GearNoTrg_last : Inport  Port=6
  Action Port : ActionPort  ActionType=case
  Bias : Bias  Bias=-1
  Bias1 : Bias  Bias=1
  Constant : Constant
  Constant1 : Constant
  Subsystem : Subsystem
  Subsystem1 : Subsystem
  Switch : Switch  Criteria=u2 ~= 0
  Switch1 : Switch  Criteria=u2 ~= 0
  Switch2 : Switch  Criteria=u2 ~= 0
  Switch3 : Switch  Criteria=u2 > Threshold
  GearNoTrg : Outport  InitialOutput=1
  wires:
  GearNo/1 -> Bias/1, Bias1/1, Subsystem/2(GearNo), Subsystem1/2(GearNo), Switch/2
  Constant/1 -> Switch/3
  Switch/1 -> GearNoTrg/1
  rotvRef/1 -> Subsystem/1(rotvRef), Subsystem1/1(rotvRef)
  Switch2/1 -> Switch/1
  Switch1/1 -> Switch2/3
  Bias/1 -> Switch1/1
  Bias1/1 -> Switch2/1
  Subsystem/1(Out1) -> Switch2/2
  Upper Limit/1 -> Subsystem/3(Upper Limit)
  nFGears/1 -> Subsystem/4(nFGears)
  Subsystem1/1(Out1) -> Switch1/2
  Lower Limit/1 -> Subsystem1/3(Lower Limit)
  Switch3/1 -> Switch1/3
  GearNoTrg_last/1 -> Switch3/2, Switch3/1
  Constant1/1 -> Switch3/3

== system PTTransmCU/CarMaker/IPG Vehicle/PowerTrain/TCU Example/TCU Example/Calculate GearNoTrg/else ==
  Action Port : ActionPort  ActionType=default
  Constant : Constant  Value=0
  GearNoTrg : Outport  InitialOutput=0
  wires:
  Constant/1 -> GearNoTrg/1

== system PTTransmCU/CarMaker/IPG Vehicle/PowerTrain/TCU Example/TCU Example/Calculate GearNoTrg/Driving/Subsystem ==
  rotvRef : Inport
  GearNo : Inport  Port=2
  Upper Limit : Inport  Port=3
  nFGears : Inport  Port=4
  Logical Operator : Logic  AllPortsSameDT=off  OutDataTypeStr=boolean
  Relational Operator1 : RelationalOperator  OutDataTypeStr=boolean
  Relational Operator2 : RelationalOperator  Operator=<  OutDataTypeStr=boolean
  Out1 : Outport
  wires:
  rotvRef/1 -> Relational Operator1/1
  Upper Limit/1 -> Relational Operator1/2
  Relational Operator1/1 -> Logical Operator/1
  Logical Operator/1 -> Out1/1
  GearNo/1 -> Relational Operator2/1
  nFGears/1 -> Relational Operator2/2
  Relational Operator2/1 -> Logical Operator/2

== system PTTransmCU/CarMaker/IPG Vehicle/PowerTrain/TCU Example/TCU Example/Calculate GearNoTrg/Driving/Subsystem1 ==
  rotvRef : Inport
  GearNo : Inport  Port=2
  Lower Limit : Inport  Port=3
  Constant : Constant
  Logical Operator : Logic  AllPortsSameDT=off  OutDataTypeStr=boolean
  Relational Operator1 : RelationalOperator  Operator=<=  OutDataTypeStr=boolean
  Relational Operator2 : RelationalOperator  Operator=>  OutDataTypeStr=boolean
  Out1 : Outport
  wires:
  rotvRef/1 -> Relational Operator1/1
  Lower Limit/1 -> Relational Operator1/2
  Relational Operator1/1 -> Logical Operator/1
  Logical Operator/1 -> Out1/1
  GearNo/1 -> Relational Operator2/1
  Constant/1 -> Relational Operator2/2
  Relational Operator2/1 -> Logical Operator/2
